simulink model "find6DOF_th"  (R2018b)
settings: Solver=ode8  StartTime=0.0  StopTime=10  FixedStep=0.01  RelTol=1e-3
undefined symbols (not defined in the file or in its folder): getVal
libraries: find6DOF_cl x1
settings Model: Creator=MAE-NCSUCORE  LastModifiedBy=MAE-NCSUCORE

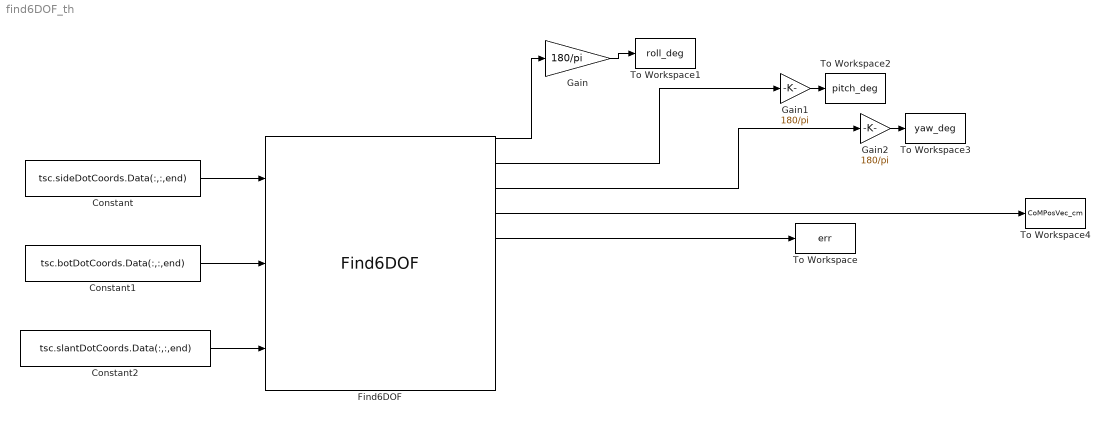
== system find6DOF_th ==
  Constant : Constant  Value=tsc.sideDotCoords.Data(:,:,end)
  Constant1 : Constant  Value=tsc.botDotCoords.Data(:,:,end)
  Constant2 : Constant  Value=tsc.slantDotCoords.Data(:,:,end)
  Find6DOF : find6DOF_cl/Find6DOF  imageDims_px=getVal('sideImageSize_px')  initialCoMPositionVec_cm=getVal('initCoMPosVec_cm')  cameraFOVAngles_deg=getVal('cameraFOV_deg')  sideEulerAngles=[0 90 90]  sideCamPositionVec_cm=getVal('sideCamPosVec_cm')  botEulerAngles=[0 180 180]  botCamPositionVec_cm=getVal('botCamPosVec_cm')  slantEulerAngles=[0 135 180]  slantCamPositionVec_cm=getVal('slntCamPosVec_cm')  sideSeparation_cm=getVal('sideDotSepDist_cm')  sidePositionVecBF_cm=[0.091 4.54 0.878]  bottomASeparation_cm=getVal('botADotSepDist_cm')  botAPositionVecBF_cm=[2.48 0 -4.53]  bottomBSeparation_cm=getVal('botBDotSepDist_cm')  botBPositionVecBG_cm=[-1 0 -4.64]
  Gain : Gain  Gain=180/pi
  Gain1 : Gain  Gain=180/pi
  Gain2 : Gain  Gain=180/pi
  To Workspace : ToWorkspace  VariableName=err  SaveFormat=Timeseries  SampleTime=-1
  To Workspace1 : ToWorkspace  VariableName=roll_deg  SaveFormat=Timeseries  SampleTime=-1
  To Workspace2 : ToWorkspace  VariableName=pitch_deg  SaveFormat=Timeseries  SampleTime=-1
  To Workspace3 : ToWorkspace  VariableName=yaw_deg  SaveFormat=Timeseries  SampleTime=-1
  To Workspace4 : ToWorkspace  VariableName=CoMPosVec_cm  SaveFormat=Timeseries  SampleTime=-1
  wires:
  Constant/1 -> Find6DOF/1
  Constant1/1 -> Find6DOF/2
  Constant2/1 -> Find6DOF/3
  Find6DOF/5 -> To Workspace/1
  Find6DOF/1 -> Gain/1
  Gain/1 -> To Workspace1/1
  Gain1/1 -> To Workspace2/1
  Gain2/1 -> To Workspace3/1
  Find6DOF/2 -> Gain1/1
  Find6DOF/3 -> Gain2/1
  Find6DOF/4 -> To Workspace4/1
